simulink model "Feedback_Configuration_1"  (R2026a)
settings: Solver=VariableStepAuto
libraries: cstblocks_lti x4
settings Model: Creator=louis  LastModifiedBy=louis

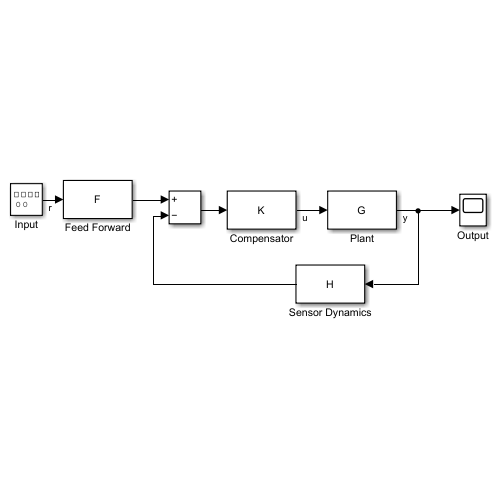
[thumbnail: Simulink's stored preview of the top-level diagram]
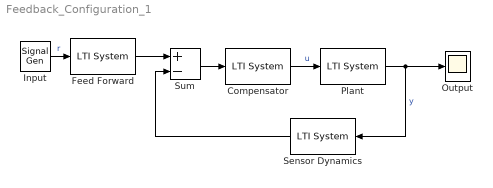
== system Feedback_Configuration_1 ==
  Compensator : cstblocks_lti/LTI System  sys=K  IC=[]  PadeOrder=0
      settings: LibrarySourceBlock=cstblocks/LTI System
  Feed Forward : cstblocks_lti/LTI System  sys=F  IC=[]  PadeOrder=0
      settings: LibrarySourceBlock=cstblocks/LTI System
  Input : SignalGenerator
  Output : Scope
  Plant : cstblocks_lti/LTI System  sys=G  IC=[]  PadeOrder=0
      settings: LibrarySourceBlock=cstblocks/LTI System
  Sensor Dynamics : cstblocks_lti/LTI System  sys=H  IC=[]  PadeOrder=0
      settings: LibrarySourceBlock=cstblocks/LTI System
  Sum : Sum  Inputs=+-
  wires:
  Input/1 -> Feed Forward/1  "r"
  Feed Forward/1 -> Sum/1
  Sensor Dynamics/1 -> Sum/2
  Sum/1 -> Compensator/1
  Compensator/1 -> Plant/1  "u"
  Plant/1 -> Output/1, Sensor Dynamics/1  "y"
